simulink model "first"  (R2019b)
settings: Solver=ode4  StartTime=0.0  StopTime=10.0  FixedStep=1e-2  RelTol=1e-3
values from neighbouring files (symbols this model uses):
  K = 1/(R*C)    (= 0.1)    [skrypt_1_4.m]    (also in skrypt_1_4_1.m = 1)
  WPC = 4    [skrypt_1_4.m]    (also in skrypt_1_4_1.m)
settings Model: Creator=marci  LastModifiedBy=marci

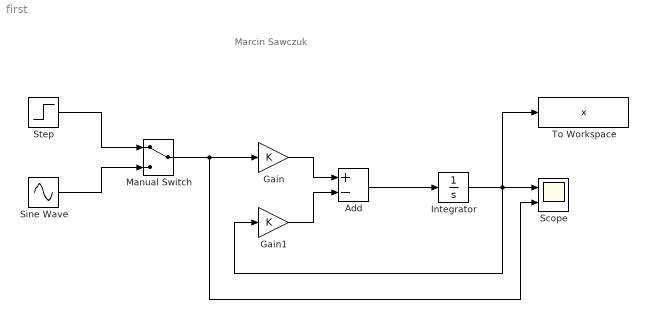
== system first ==
  note: Marcin Sawczuk
  Add : Sum  Inputs=+-
  Gain : Gain  Gain=K
  Gain1 : Gain  Gain=K
  Integrator : Integrator  InitialCondition=WPC
  Manual Switch : ManualSwitch
  Scope : Scope  NumInputPorts=2
  Sine Wave : Sin  Frequency=2*pi*10  SampleTime=0
  Step : Step  After=2  SampleTime=0
  To Workspace : ToWorkspace  VariableName=x  SampleTime=-1
      settings: Save2DSignal=2-D array (concatenate along first dimension)
  wires:
  Step/1 -> Manual Switch/1
  Sine Wave/1 -> Manual Switch/2
  Manual Switch/1 -> Scope/2, Gain/1
  Gain/1 -> Add/1
  Gain1/1 -> Add/2
  Add/1 -> Integrator/1
  Integrator/1 -> Gain1/1, To Workspace/1, Scope/1
